simulink model "Realimentador_SIM"  (R2018a)
settings: Solver=FixedStepAuto  StartTime=0.0  StopTime=500E-6  FixedStep=1E-9  RelTol=1e-3
libraries: powerlib_meascontrol x2
settings Model: Creator=emanu  LastModifiedBy=Ema

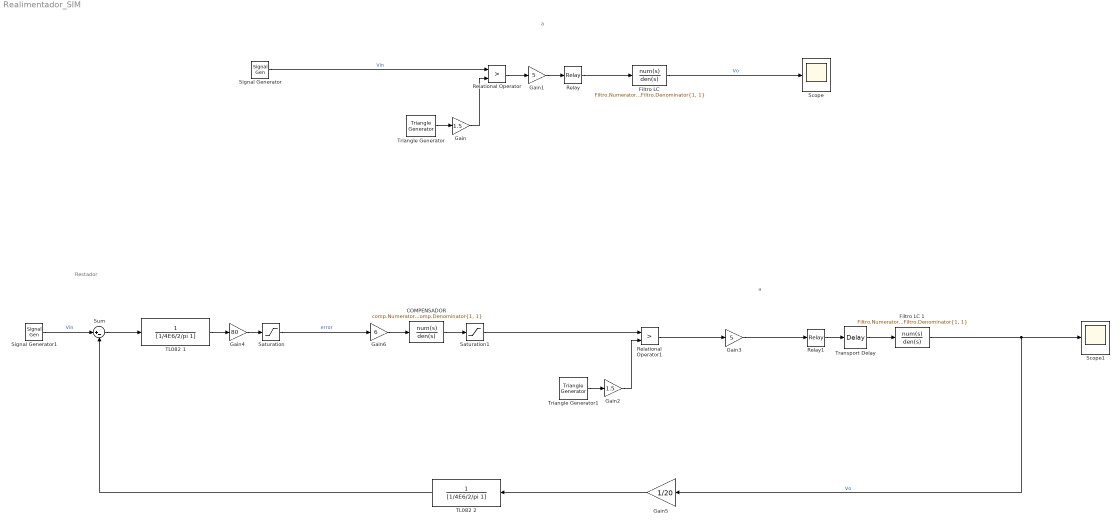
== system Realimentador_SIM ==
  note: Restador
  note: a
  note: a
  COMPENSADOR : TransferFcn  Numerator=comp.Numerator{1, 1}  Denominator=comp.Denominator{1, 1}
  "Filtro LC " : TransferFcn  Numerator=Filtro.Numerator{1, 1}  Denominator=Filtro.Denominator{1, 1}
  Filtro LC 1 : TransferFcn  Numerator=Filtro.Numerator{1, 1}  Denominator=Filtro.Denominator{1, 1}
  Gain : Gain  Gain=1.5
  Gain1 : Gain  Gain=5
  Gain2 : Gain  Gain=1.5
  Gain3 : Gain  Gain=5
  Gain4 : Gain  Gain=80
  Gain5 : Gain  Gain=1/20
  Gain6 : Gain  Gain=6
  Relational Operator : RelationalOperator  Operator=>  OutDataTypeStr=boolean  RndMeth=Simplest
  Relational Operator1 : RelationalOperator  Operator=>  OutDataTypeStr=boolean  RndMeth=Simplest
  Relay : Relay  OnSwitchValue=1  OffSwitchValue=1  OnOutputValue=30  OffOutputValue=-30  OutDataTypeStr=double
  Relay1 : Relay  OnSwitchValue=1  OffSwitchValue=1  OnOutputValue=30  OffOutputValue=-30  OutDataTypeStr=double
  Saturation : Saturate  UpperLimit=13  LowerLimit=-13
  Saturation1 : Saturate  UpperLimit=13  LowerLimit=-13
  Scope : Scope
  Scope1 : Scope
  Signal Generator : SignalGenerator  Amplitude=1.1  Frequency=20E3
  Signal Generator1 : SignalGenerator  Amplitude=1.1  Frequency=20E3
  Sum : Sum  Inputs=|+-
  TL082 1 : TransferFcn  Denominator=[1/4E6/2/pi 1]
  TL082 2 : TransferFcn  Denominator=[1/4E6/2/pi 1]
  Transport Delay : TransportDelay  DelayTime=200E-9
  Triangle Generator : powerlib_meascontrol/Pulse & Signal Generators/Triangle Generator  Freq=200E3  Phase=90  Ts=0
  Triangle Generator1 : powerlib_meascontrol/Pulse & Signal Generators/Triangle Generator  Freq=200E3  Phase=90  Ts=0
  wires:
  Triangle Generator/1 -> Gain/1
  Signal Generator/1 -> Relational Operator/1  "Vin"
  Gain/1 -> Relational Operator/2
  Relational Operator/1 -> Gain1/1
  Gain1/1 -> Relay/1
  Relay/1 -> "Filtro LC "/1
  "Filtro LC "/1 -> Scope/1  "Vo"
  Filtro LC 1/1 -> Gain5/1, Scope1/1  "Vo"
  Gain3/1 -> Relay1/1
  Gain2/1 -> Relational Operator1/2
  Triangle Generator1/1 -> Gain2/1
  Signal Generator1/1 -> Sum/1  "Vin"
  Relay1/1 -> Transport Delay/1
  Relational Operator1/1 -> Gain3/1
  Gain4/1 -> Saturation/1
  Gain5/1 -> TL082 2/1
  Sum/1 -> TL082 1/1
  Transport Delay/1 -> Filtro LC 1/1
  TL082 1/1 -> Gain4/1
  Gain6/1 -> COMPENSADOR/1
  COMPENSADOR/1 -> Saturation1/1
  Saturation/1 -> Gain6/1  "error"
  Saturation1/1 -> Relational Operator1/1
  TL082 2/1 -> Sum/2
